simulink model "kalman_gyro_synchronous"  (R2014a)
settings: Solver=FixedStepDiscrete  StartTime=0.0  StopTime=t_sim  FixedStep=t_step  RelTol=1e-3
undefined symbols (not defined in the file): omega_B
libraries: lib_gyro_fusion x10
settings Model: Creator=kirill  LastModifiedBy=kirill

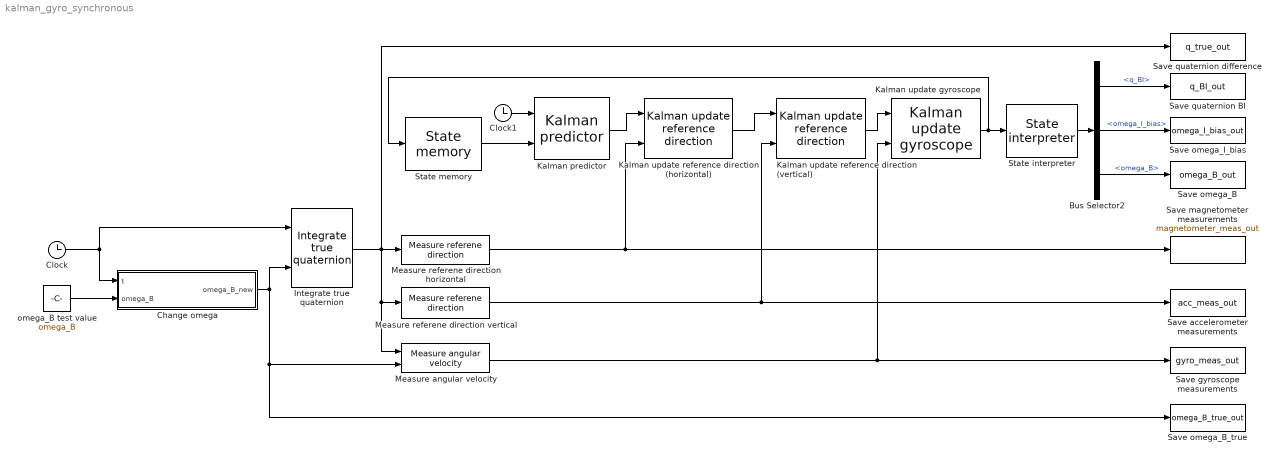
== system kalman_gyro_synchronous ==
  Bus Selector2 : BusSelector  OutputSignals=q_BI,omega_I_bias,omega_B
  Change omega : MATLAB Function  TreatAsAtomicUnit=on
  Clock : Clock
  Clock1 : Clock
  Integrate true quaternion : lib_gyro_fusion/Integrate true quaternion  q_BI_init=q_init
  Kalman predictor : lib_gyro_fusion/Kalman predictor  q_noise=q_noise  omega_B_noise=omega_B_noise  omega_I_bias_noise=omega_bias_I_noise
  Kalman update gyroscope : lib_gyro_fusion/Kalman update gyroscope
  Kalman update reference direction (horizontal) : lib_gyro_fusion/Kalman update reference direction
  Kalman update reference direction (vertical) : lib_gyro_fusion/Kalman update reference direction
  Measure angular velocity : lib_gyro_fusion/Measure angular velocity
  Measure referene direction horizontal : lib_gyro_fusion/Measure referene direction  ref_direction=horizontal_direction  measurement_noise_power=horizontal_direction_noise_power  measurement_sample_rate=t_step  source_seeds=horizontal_direction_seeds  R_direction=horizontal_direction_R
  Measure referene direction vertical : lib_gyro_fusion/Measure referene direction  ref_direction=vertical_direction  measurement_noise_power=vertical_direction_noise_power  measurement_sample_rate=t_step  source_seeds=vertical_direction_seeds  R_direction=vertical_direction_R
  Save accelerometer measurements : ToWorkspace  VariableName=acc_meas_out  SaveFormat=Timeseries  SampleTime=-1
  Save gyroscope measurements : ToWorkspace  VariableName=gyro_meas_out  SaveFormat=Timeseries  SampleTime=-1
  Save magnetometer measurements : ToWorkspace  VariableName=magnetometer_meas_out  SaveFormat=Timeseries  SampleTime=-1
  Save omega_B : ToWorkspace  VariableName=omega_B_out  SaveFormat=Timeseries  SampleTime=-1
  Save omega_B_true : ToWorkspace  VariableName=omega_B_true_out  SaveFormat=Timeseries  SampleTime=-1
  Save omega_I_bias : ToWorkspace  VariableName=omega_I_bias_out  SaveFormat=Timeseries  SampleTime=-1
  Save quaternion BI : ToWorkspace  VariableName=q_BI_out  SaveFormat=Timeseries  SampleTime=-1
  Save quaternion difference : ToWorkspace  VariableName=q_true_out  SaveFormat=Timeseries  SampleTime=-1
  State interpreter : lib_gyro_fusion/State interpreter
  State memory : lib_gyro_fusion/State memory  q_BI_init=[1; 0; 0; 0]  omega_B_init=[0; 0; 0]  omega_I_bias_init=[0; 0; 0]  P_full_init=eye(9)
  omega_B test value : Constant  Value=omega_B
  wires:
  State memory/1 -> Kalman predictor/2
  Clock/1 -> Change omega/1(t), Integrate true quaternion/1
  Integrate true quaternion/1 -> Save quaternion difference/1, Measure angular velocity/1, Measure referene direction vertical/1, Measure referene direction horizontal/1
  Bus Selector2/2 -> Save omega_I_bias/1  "<omega_I_bias>"
  Bus Selector2/1 -> Save quaternion BI/1  "<q_BI>"
  Clock1/1 -> Kalman predictor/1
  Kalman predictor/1 -> Kalman update reference direction (horizontal)/1
  Measure referene direction horizontal/1 -> Save magnetometer measurements/1, Kalman update reference direction (horizontal)/2
  Measure referene direction vertical/1 -> Kalman update reference direction (vertical)/2, Save accelerometer measurements/1
  Change omega/1(omega_B_new) -> Integrate true quaternion/2, Save omega_B_true/1, Measure angular velocity/2
  omega_B test value/1 -> Change omega/2(omega_B)
  Kalman update gyroscope/1 -> State interpreter/1, State memory/1
  Measure angular velocity/1 -> Save gyroscope measurements/1, Kalman update gyroscope/2
  Bus Selector2/3 -> Save omega_B/1  "<omega_B>"
  State interpreter/1 -> Bus Selector2/1
  Kalman update reference direction (horizontal)/1 -> Kalman update reference direction (vertical)/1
  Kalman update reference direction (vertical)/1 -> Kalman update gyroscope/1

== matlab function kalman_gyro_synchronous/Change omega ==
  data: t input; omega_B input; omega_B_new output
function omega_B_new = change_omega(t, omega_B)
%#codegen
a = [cos(2 * pi * t / 120); cos(2 * pi * t / 20.5); cos(2 * pi * t / 81.5)];
omega_B_new = a.* omega_B;
